simulink model "syteme"  (R2022b)
settings: Solver=VariableStepAuto  StartTime=0.0  StopTime=700  RelTol=1e-3
values from neighbouring files (symbols this model uses):
  A = [-1/T1     0  A3/(A1*T1)           0 ... (first row only)    [scriptm.m]
  a1 = 71e-3    (= 0.071)    [scriptm.m]
  A1 = 28    [scriptm.m]
  A2 = 32    [scriptm.m]
  a2 = 57e-3    (= 0.057)    [scriptm.m]
  A3 = A1    (= 28)    [scriptm.m]
  a3 = a1    (= 0.071)    [scriptm.m]
  A4 = A2    (= 32)    [scriptm.m]
  a4 = a2    (= 0.057)    [scriptm.m]
  B = [ (gamma1*k1)/A1                 0 ... (first row only)    [scriptm.m]
  C = [1 0 0 0 ... (first row only)    [scriptm.m]
  D = [0 0 ... (first row only)    [scriptm.m]
  g = 981    [scriptm.m]
  gamma1 = 0.7    [scriptm.m]
  gamma2 = 0.6    [scriptm.m]
  k1 = 3.33    [scriptm.m]
  k2 = 3.35    [scriptm.m]
  v1_0 = 3    [scriptm.m]
  v2_0 = 3    [scriptm.m]
settings Model: Creator=driss  LastModifiedBy=driss

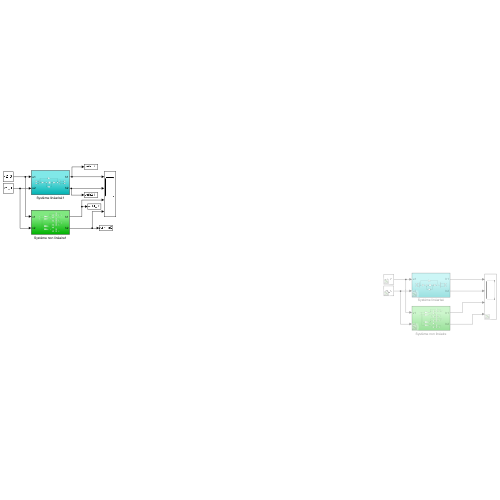
[thumbnail: Simulink's stored preview of the top-level diagram]
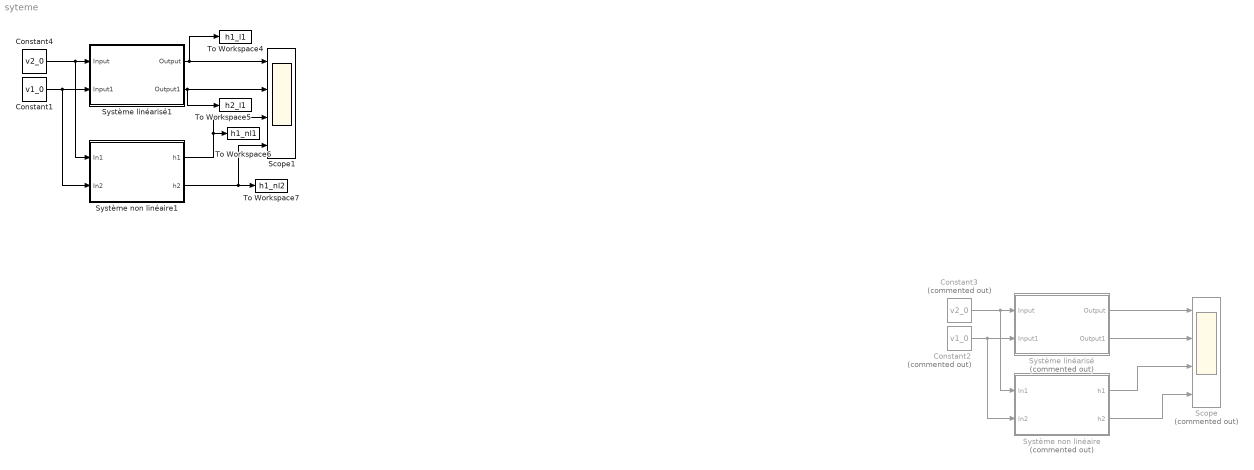
== system syteme ==
  Constant1 : Constant  Value=v1_0
  Constant2 : Constant  Commented=on  Value=v1_0
  Constant3 : Constant  Commented=on  Value=v2_0
  Constant4 : Constant  Value=v2_0
  Scope : Scope  Commented=on  NumInputPorts=4
  Scope1 : Scope  NumInputPorts=4
  Système linéarisé : Subsystem  Commented=on
  Système linéarisé1 : Subsystem
  Système non linéaire : Subsystem  Commented=on
  Système non linéaire1 : Subsystem
  To Workspace4 : ToWorkspace  VariableName=h1_l1  SaveFormat=Timeseries  SampleTime=-1
  To Workspace5 : ToWorkspace  VariableName=h2_l1  SaveFormat=Timeseries  SampleTime=-1
  To Workspace6 : ToWorkspace  VariableName=h1_nl1  SaveFormat=Timeseries  SampleTime=-1
  To Workspace7 : ToWorkspace  VariableName=h1_nl2  SaveFormat=Timeseries  SampleTime=-1
  wires:
  Système linéarisé/1(Output) -> Scope/1
  Constant3/1 -> Système non linéaire/1(In1), Système linéarisé/1(Input)
  Constant2/1 -> Système linéarisé/2(Input1), Système non linéaire/2(In2)
  Système non linéaire/1(h1) -> Scope/3
  Système non linéaire/2(h2) -> Scope/4
  Système linéarisé/2(Output1) -> Scope/2
  Système non linéaire1/2(h2) -> To Workspace7/1, Scope1/4
  Constant1/1 -> Système linéarisé1/2(Input1), Système non linéaire1/2(In2)
  Système non linéaire1/1(h1) -> Scope1/3, To Workspace6/1
  Constant4/1 -> Système non linéaire1/1(In1), Système linéarisé1/1(Input)
  Système linéarisé1/1(Output) -> To Workspace4/1, Scope1/1
  Système linéarisé1/2(Output1) -> To Workspace5/1, Scope1/2

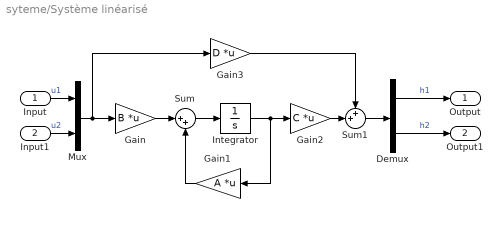
== system syteme/Système linéarisé ==
  Input : Inport
  Input1 : Inport  Port=2
  Demux : Demux  Outputs=2
  Gain : Gain  Gain=B  Multiplication=Matrix(K*u)
  Gain1 : Gain  Gain=A  Multiplication=Matrix(K*u)
  Gain2 : Gain  Gain=C  Multiplication=Matrix(K*u)
  Gain3 : Gain  Gain=D  Multiplication=Matrix(K*u)
  Integrator : Integrator
  Mux : Mux  Inputs=2
  Sum : Sum  Inputs=|++
  Sum1 : Sum  Inputs=++|
  Output : Outport
  Output1 : Outport  Port=2
  wires:
  Gain2/1 -> Sum1/2
  Integrator/1 -> Gain2/1, Gain1/1
  Gain3/1 -> Sum1/1
  Sum1/1 -> Demux/1
  Sum/1 -> Integrator/1
  Gain/1 -> Sum/1
  Gain1/1 -> Sum/2
  Mux/1 -> Gain3/1, Gain/1
  Input/1 -> Mux/1  "u1"
  Input1/1 -> Mux/2  "u2"
  Demux/1 -> Output/1  "h1"
  Demux/2 -> Output1/1  "h2"

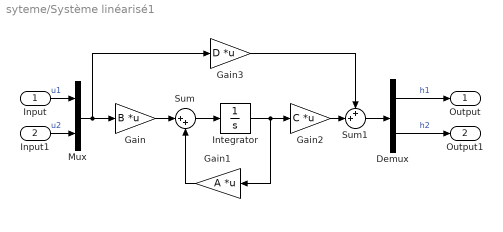
== system syteme/Système linéarisé1 ==
  Input : Inport
  Input1 : Inport  Port=2
  Demux : Demux  Outputs=2
  Gain : Gain  Gain=B  Multiplication=Matrix(K*u)
  Gain1 : Gain  Gain=A  Multiplication=Matrix(K*u)
  Gain2 : Gain  Gain=C  Multiplication=Matrix(K*u)
  Gain3 : Gain  Gain=D  Multiplication=Matrix(K*u)
  Integrator : Integrator
  Mux : Mux  Inputs=2
  Sum : Sum  Inputs=|++
  Sum1 : Sum  Inputs=++|
  Output : Outport
  Output1 : Outport  Port=2
  wires:
  Gain2/1 -> Sum1/2
  Integrator/1 -> Gain2/1, Gain1/1
  Gain3/1 -> Sum1/1
  Sum1/1 -> Demux/1
  Sum/1 -> Integrator/1
  Gain/1 -> Sum/1
  Gain1/1 -> Sum/2
  Mux/1 -> Gain3/1, Gain/1
  Input/1 -> Mux/1  "u1"
  Input1/1 -> Mux/2  "u2"
  Demux/1 -> Output/1  "h1"
  Demux/2 -> Output1/1  "h2"

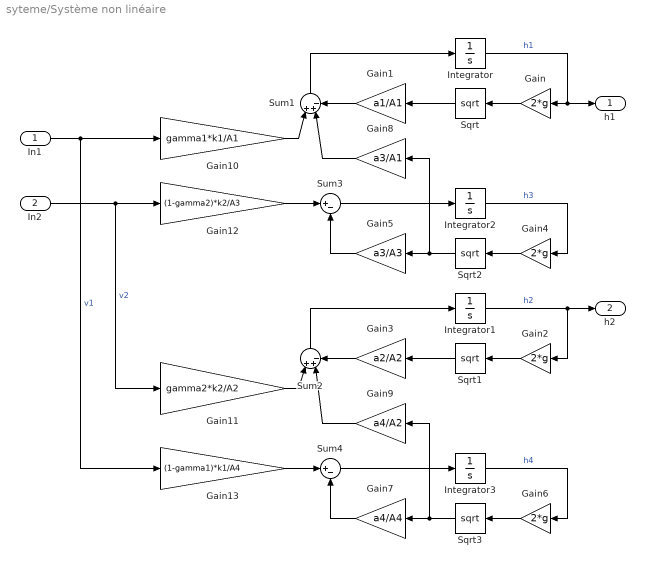
== system syteme/Système non linéaire ==
  In1 : Inport
  In2 : Inport  Port=2
  Gain{,2,4,6} (4 alike) : Gain  Gain=2*g
  Gain1 : Gain  Gain=a1/A1
  Gain10 : Gain  Gain=gamma1*k1/A1
  Gain11 : Gain  Gain=gamma2*k2/A2
  Gain12 : Gain  Gain=(1-gamma2)*k2/A3
  Gain13 : Gain  Gain=(1-gamma1)*k1/A4
  Gain3 : Gain  Gain=a2/A2
  Gain5 : Gain  Gain=a3/A3
  Gain7 : Gain  Gain=a4/A4
  Gain8 : Gain  Gain=a3/A1
  Gain9 : Gain  Gain=a4/A2
  Integrator{,1..3} (4 alike) : Integrator
  Sqrt{,1..3} (4 alike) : Sqrt
  Sum1 : Sum  Inputs=|++-
  Sum2 : Sum  Inputs=|++-
  Sum3 : Sum  Inputs=|+-
  Sum4 : Sum  Inputs=|+-
  h1 : Outport
  h2 : Outport  Port=2
  wires:
  Gain6/1 -> Sqrt3/1
  Sqrt1/1 -> Gain3/1
  Gain9/1 -> Sum2/2
  Gain10/1 -> Sum1/1
  Integrator/1 -> h1/1, Gain/1  "h1"
  Gain4/1 -> Sqrt2/1
  Sum2/1 -> Integrator1/1
  Gain3/1 -> Sum2/3
  Sqrt2/1 -> Gain8/1, Gain5/1
  Sqrt/1 -> Gain1/1
  Sqrt3/1 -> Gain9/1, Gain7/1
  Gain7/1 -> Sum4/2
  Gain8/1 -> Sum1/2
  Gain12/1 -> Sum3/1
  Gain13/1 -> Sum4/1
  In2/1 -> Gain11/1, Gain12/1  "v2"
  Integrator2/1 -> Gain4/1  "h3"
  Gain5/1 -> Sum3/2
  Gain/1 -> Sqrt/1
  Gain11/1 -> Sum2/1
  Sum1/1 -> Integrator/1
  In1/1 -> Gain13/1, Gain10/1  "v1"
  Integrator1/1 -> h2/1, Gain2/1  "h2"
  Gain2/1 -> Sqrt1/1
  Sum3/1 -> Integrator2/1
  Gain1/1 -> Sum1/3
  Integrator3/1 -> Gain6/1  "h4"
  Sum4/1 -> Integrator3/1

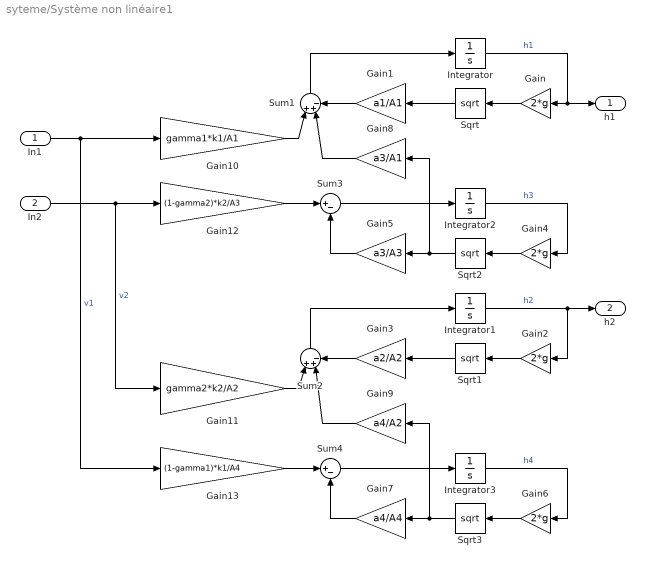
== system syteme/Système non linéaire1 ==
  In1 : Inport
  In2 : Inport  Port=2
  Gain{,2,4,6} (4 alike) : Gain  Gain=2*g
  Gain1 : Gain  Gain=a1/A1
  Gain10 : Gain  Gain=gamma1*k1/A1
  Gain11 : Gain  Gain=gamma2*k2/A2
  Gain12 : Gain  Gain=(1-gamma2)*k2/A3
  Gain13 : Gain  Gain=(1-gamma1)*k1/A4
  Gain3 : Gain  Gain=a2/A2
  Gain5 : Gain  Gain=a3/A3
  Gain7 : Gain  Gain=a4/A4
  Gain8 : Gain  Gain=a3/A1
  Gain9 : Gain  Gain=a4/A2
  Integrator{,1..3} (4 alike) : Integrator
  Sqrt{,1..3} (4 alike) : Sqrt
  Sum1 : Sum  Inputs=|++-
  Sum2 : Sum  Inputs=|++-
  Sum3 : Sum  Inputs=|+-
  Sum4 : Sum  Inputs=|+-
  h1 : Outport
  h2 : Outport  Port=2
  wires:
  Gain6/1 -> Sqrt3/1
  Sqrt1/1 -> Gain3/1
  Gain9/1 -> Sum2/2
  Gain10/1 -> Sum1/1
  Integrator/1 -> h1/1, Gain/1  "h1"
  Gain4/1 -> Sqrt2/1
  Sum2/1 -> Integrator1/1
  Gain3/1 -> Sum2/3
  Sqrt2/1 -> Gain8/1, Gain5/1
  Sqrt/1 -> Gain1/1
  Sqrt3/1 -> Gain9/1, Gain7/1
  Gain7/1 -> Sum4/2
  Gain8/1 -> Sum1/2
  Gain12/1 -> Sum3/1
  Gain13/1 -> Sum4/1
  In2/1 -> Gain11/1, Gain12/1  "v2"
  Integrator2/1 -> Gain4/1  "h3"
  Gain5/1 -> Sum3/2
  Gain/1 -> Sqrt/1
  Gain11/1 -> Sum2/1
  Sum1/1 -> Integrator/1
  In1/1 -> Gain13/1, Gain10/1  "v1"
  Integrator1/1 -> h2/1, Gain2/1  "h2"
  Gain2/1 -> Sqrt1/1
  Sum3/1 -> Integrator2/1
  Gain1/1 -> Sum1/3
  Integrator3/1 -> Gain6/1  "h4"
  Sum4/1 -> Integrator3/1
